simulink model "FirstOrder_Sim"  (R2022b)
settings: Solver=VariableStepAuto  StartTime=0.0  StopTime=10.0  RelTol=1e-3
settings Model: Creator=MAAM  LastModifiedBy=MAAM

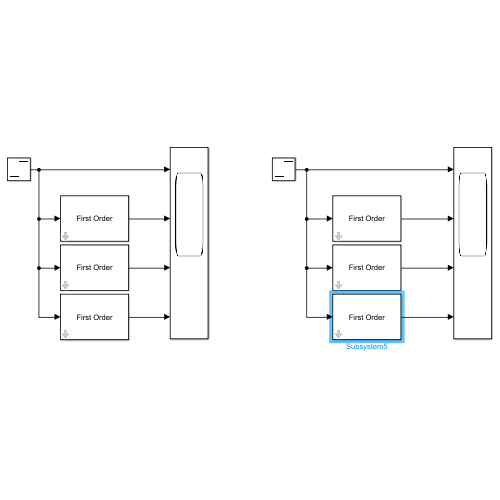
[thumbnail: Simulink's stored preview of the top-level diagram]
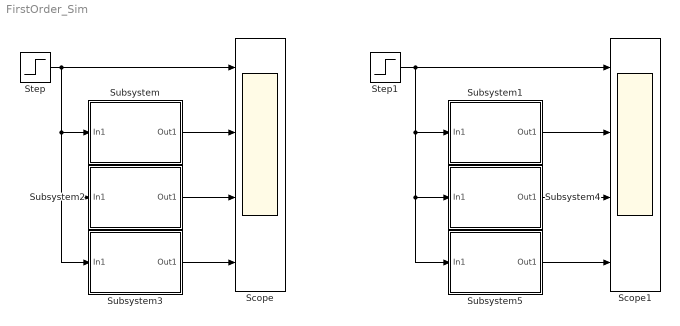
== system FirstOrder_Sim ==
  Scope : Scope  NumInputPorts=4
  Scope1 : Scope  NumInputPorts=4
  Step : Step  SampleTime=0
  Step1 : Step  SampleTime=0
  Subsystem : Subsystem  mask{T=0.25, K=1}
      mask prompts: T "Time Constant "T""; K "Gain "K""
      mask Display: fprintf("First Order");
  Subsystem1 : Subsystem  mask{T=0.25, K=0.5}
      mask prompts: T "Time Constant "T""; K "Gain "K""
      mask Display: fprintf("First Order");
  Subsystem2 : Subsystem  mask{T=0.5, K=1}
      mask prompts: T "Time Constant "T""; K "Gain "K""
      mask Display: fprintf("First Order");
  Subsystem3 : Subsystem  mask{T=1, K=1}
      mask prompts: T "Time Constant "T""; K "Gain "K""
      mask Display: fprintf("First Order");
  Subsystem4 : Subsystem  mask{T=0.25, K=1}
      mask prompts: T "Time Constant "T""; K "Gain "K""
      mask Display: fprintf("First Order");
  Subsystem5 : Subsystem  mask{T=0.25, K=1.5}
      mask prompts: T "Time Constant "T""; K "Gain "K""
      mask Display: fprintf("First Order");
  wires:
  Step/1 -> Subsystem/1(In1), Subsystem2/1(In1), Subsystem3/1(In1), Scope/1
  Subsystem/1(Out1) -> Scope/2
  Subsystem2/1(Out1) -> Scope/3
  Subsystem3/1(Out1) -> Scope/4
  Subsystem4/1(Out1) -> Scope1/3
  Subsystem5/1(Out1) -> Scope1/4
  Subsystem1/1(Out1) -> Scope1/2
  Step1/1 -> Subsystem1/1(In1), Subsystem4/1(In1), Subsystem5/1(In1), Scope1/1

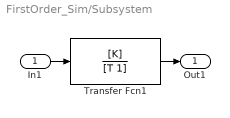
== system FirstOrder_Sim/Subsystem ==
  In1 : Inport
  Transfer Fcn1 : TransferFcn  Numerator=[K]  Denominator=[T 1]
  Out1 : Outport
  wires:
  Transfer Fcn1/1 -> Out1/1
  In1/1 -> Transfer Fcn1/1

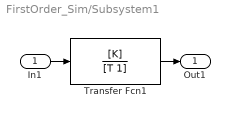
== system FirstOrder_Sim/Subsystem1 ==
  In1 : Inport
  Transfer Fcn1 : TransferFcn  Numerator=[K]  Denominator=[T 1]
  Out1 : Outport
  wires:
  In1/1 -> Transfer Fcn1/1
  Transfer Fcn1/1 -> Out1/1

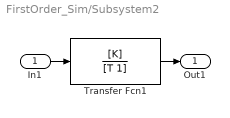
== system FirstOrder_Sim/Subsystem2 ==
  In1 : Inport
  Transfer Fcn1 : TransferFcn  Numerator=[K]  Denominator=[T 1]
  Out1 : Outport
  wires:
  In1/1 -> Transfer Fcn1/1
  Transfer Fcn1/1 -> Out1/1

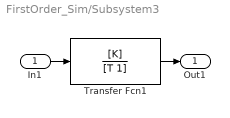
== system FirstOrder_Sim/Subsystem3 ==
  In1 : Inport
  Transfer Fcn1 : TransferFcn  Numerator=[K]  Denominator=[T 1]
  Out1 : Outport
  wires:
  Transfer Fcn1/1 -> Out1/1
  In1/1 -> Transfer Fcn1/1

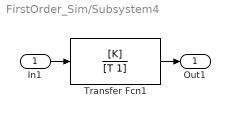
== system FirstOrder_Sim/Subsystem4 ==
  In1 : Inport
  Transfer Fcn1 : TransferFcn  Numerator=[K]  Denominator=[T 1]
  Out1 : Outport
  wires:
  Transfer Fcn1/1 -> Out1/1
  In1/1 -> Transfer Fcn1/1

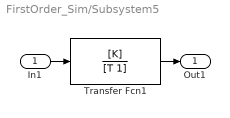
== system FirstOrder_Sim/Subsystem5 ==
  In1 : Inport
  Transfer Fcn1 : TransferFcn  Numerator=[K]  Denominator=[T 1]
  Out1 : Outport
  wires:
  In1/1 -> Transfer Fcn1/1
  Transfer Fcn1/1 -> Out1/1
